simulink model "pwm_ppm"  (R2020a)
settings: Solver=VariableStepAuto  StartTime=0.0  StopTime=10.0  RelTol=1e-3
libraries: powerlib_meascontrol x2, simulink x1
settings Model: Creator=91735  LastModifiedBy=91735

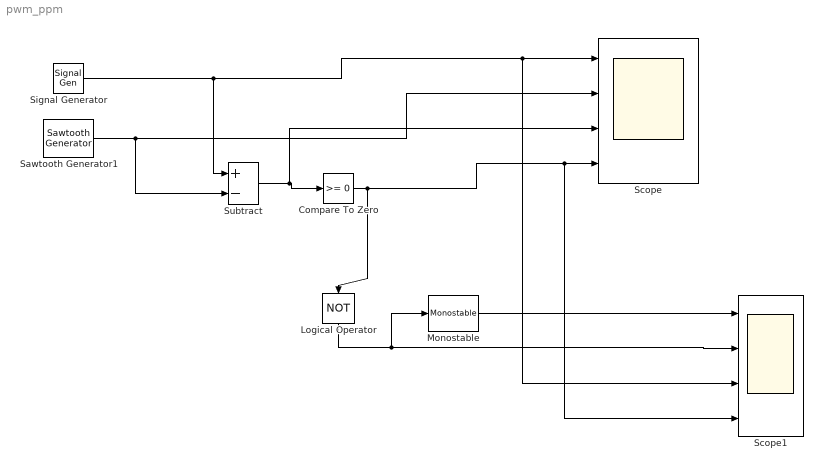
== system pwm_ppm ==
  Compare To Zero : simulink/Logic and Bit Operations/Compare To Zero  relop=>=  OutDataTypeStr=boolean
  Logical Operator : Logic  Operator=NOT  IconShape=distinctive  AllPortsSameDT=off  OutDataTypeStr=boolean
  Monostable : powerlib_meascontrol/Logic/Monostable  EdgeDetect=Rising  PulseDuration=0.05  ic=0  Ts=0
      settings: SourceProductBaseCode=PS
  Sawtooth Generator1 : powerlib_meascontrol/Pulse & Signal Generators/Sawtooth Generator  Freq=1e3  Phase=180  Ts=0
  Scope : Scope  NumInputPorts=4
  Scope1 : Scope  NumInputPorts=4
  Signal Generator : SignalGenerator  Amplitude=.9  Units=rad/sec
  Subtract : Sum  Inputs=+-
  wires:
  Signal Generator/1 -> Subtract/1, Scope1/3, Scope/1
  Sawtooth Generator1/1 -> Subtract/2, Scope/2
  Subtract/1 -> Scope/3, Compare To Zero/1
  Compare To Zero/1 -> Logical Operator/1, Scope1/4, Scope/4
  Logical Operator/1 -> Scope1/2, Monostable/1
  Monostable/1 -> Scope1/1
